simulink model "Lab2Task3"  (R2016a)
settings: Solver=VariableStepAuto  StartTime=0.0  StopTime=150.0  RelTol=1e-3
settings Model: Creator=Thomas  LastModifiedBy=Thomas

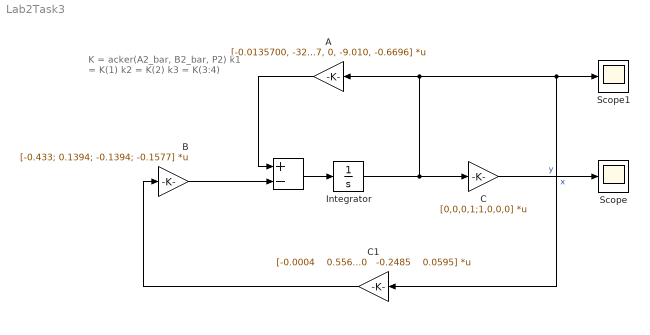
== system Lab2Task3 ==
  note: K = acker(A2_bar, B2_bar, P2)
      | k1 = K(1)
      | k2 = K(2)
      | k3 = K(3:4)
  "   " : Sum  Inputs=+-
  A : Gain  Gain=[-0.0135700, -32.3, -46.3, 0; 0.0001200, 0, 1.214, 0; -0.0001212, 0, -1.214, 1;0.00057, 0, -9.010, -0.6696]  Multiplication=Matrix(K*u)
  B : Gain  Gain=[-0.433; 0.1394; -0.1394; -0.1577]  Multiplication=Matrix(K*u)
  C : Gain  Gain=[0,0,0,1;1,0,0,0]  Multiplication=Matrix(K*u)
  C1 : Gain  Gain="[-0.0004    0.5560   -0.2485    0.0595]"  Multiplication=Matrix(K*u)
  Integrator : Integrator  InitialCondition=[100; 0; 0.2; 0]
  Scope : Scope
  Scope1 : Scope
  wires:
  "   "/1 -> Integrator/1
  A/1 -> "   "/1
  B/1 -> "   "/2
  Integrator/1 -> A/1, C1/1, Scope1/1, C/1  "x"
  C/1 -> Scope/1  "y"
  C1/1 -> B/1
